simulink model "TCPIPmatlab"  (R2018b)
settings: Solver=VariableStepAuto  StartTime=0.0  StopTime=10.0  MaxStep=0.0001  MinStep=0.0001  RelTol=1e-3
undefined symbols (not defined in the file): f
libraries: instrumentlib x2
settings Model: Creator=c8501009  LastModifiedBy=c8501009
settings DataIOCC: ReturnWorkspaceOutputs=on

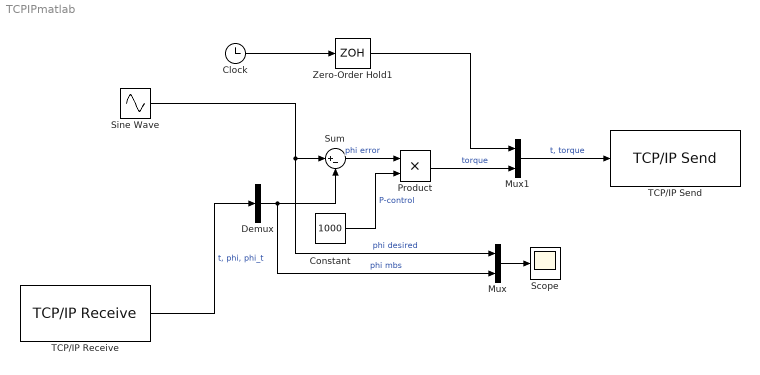
== system TCPIPmatlab ==
  Clock : Clock
  Constant : Constant  Value=1000  SampleTime=0.01
  Demux : Demux  Outputs=3
  Mux : Mux  Inputs=2
  Mux1 : Mux  Inputs=2
  Product : Product
  Scope : Scope
  Sine Wave : Sin  Amplitude=0.5*pi  Bias=-0.5*pi  Frequency=0.2*pi*2  Phase=0.5*pi  SampleTime=0.01
  Sum : Sum  Inputs=|+-
  TCP/IP Receive : instrumentlib/TCP//IP Receive  Priority=1  Host=127.0.0.1  Port=52421  DataSize=3  EnableBlockingMode=on  Timeout=2  SampleTime=0.01  DataType=double  ByteOrder=BigEndian  ASCIIFormatting=%f,  Terminator=LF
  TCP/IP Send : instrumentlib/TCP//IP Send  Priority=2  Host=127.0.0.1  Port=52421  EnableBlockingMode=off  Timeout=10  ByteOrder=BigEndian  TransferDelay=on
  Zero-Order Hold1 : ZeroOrderHold  SampleTime=-1
  wires:
  TCP/IP Receive/1 -> Demux/1  "t, phi, phi_t"
  Mux/1 -> Scope/1
  Clock/1 -> Zero-Order Hold1/1
  Zero-Order Hold1/1 -> Mux1/1
  Mux1/1 -> TCP/IP Send/1  "t, torque"
  Sine Wave/1 -> Mux/1, Sum/1  "phi desired"
  Demux/2 -> Mux/2, Sum/2  "phi mbs"
  Product/1 -> Mux1/2  "torque"
  Sum/1 -> Product/1  "phi error"
  Constant/1 -> Product/2  "P-control"
